simulink model "Problem8"  (R2020b)
settings: Solver=VariableStepAuto  StartTime=0.0  StopTime=inf  RelTol=1e-3
settings Model: EnablePacing=on  PacingRate=0.089000  Creator=ASUS  LastModifiedBy=ASUS

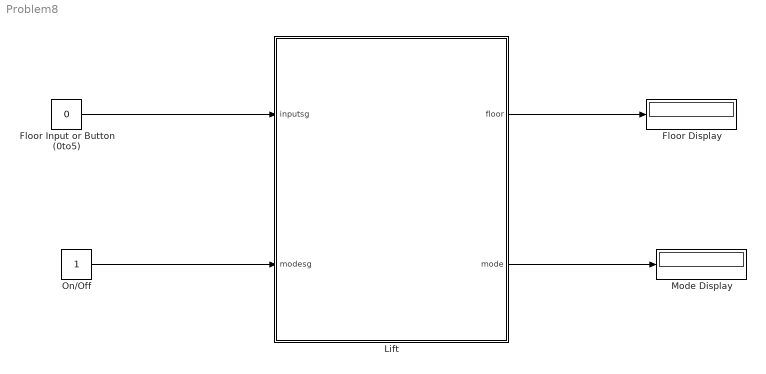
== system Problem8 ==
  Floor Display : Display
  Floor Input or Button (0to5) : Constant  Value=0
  "Lift " : Stateflow chart  TreatAsAtomicUnit=on
  Mode Display : Display
  On/Off : Constant
  wires:
  "Lift "/1(floor) -> Floor Display/1
  Floor Input or Button (0to5)/1 -> "Lift "/1(inputsg)
  "Lift "/2(mode) -> Mode Display/1
  On/Off/1 -> "Lift "/2(modesg)

== stateflow chart Problem8/Lift  ==
  state Floormovement(Floor) [function]
    (default) -> (junction 97)
    (junction 97) -> (junction 107) [order 3] : [inputsg<Floor]{send(DOWN);}
    (junction 97) -> (junction 100) [order 1] : [inputsg>Floor]{send(UP);}
    (junction 107) -> (junction 109)
    (junction 97) -> (junction 104) [order 2] : [inputsg==Floor]
    (junction 100) -> (junction 102)
    (junction 109) -> (junction 104)
    (junction 102) -> (junction 104)
    (junction 104) -> (junction 113)
  state Lift_Working_Operation [parallel]
    entry:
    mode=0;
    settings: executionOrder=1
    state LiftOn
      state Floor2
        en:
        mode=1;
        du:
        floor=2;
        Floormovement(floor);
        exit:
        mode=0
      state GroundFloor
        en:
        mode=1;
        du:
        floor=0;
        Floormovement(floor);
        exit:
        mode=0;
      state Floor1
        en:
        mode=1;
        du:
        floor=1;
        Floormovement(floor);
        exit:
        mode=0
      state Floor3
        en:
        mode=1;
        du:
        floor=3;
        Floormovement(floor);
        exit:
        mode=0
      state Floor4
        en:
        mode=1;
        du:
        floor=4;
        Floormovement(floor);
        exit:
        mode=0
      state Floor5
        en:
        mode=1;
        du:
        floor=5;
        Floormovement(floor);
        exit:
        mode=0
      (default) -> GroundFloor
      GroundFloor -> Floor1 : UP
      Floor2 -> Floor3 [order 1] : UP
      Floor1 -> Floor2 [order 1] : UP
      Floor3 -> Floor4 [order 1] : UP
      Floor4 -> Floor5 [order 1] : UP
      Floor1 -> GroundFloor [order 2] : DOWN
      Floor2 -> Floor1 [order 2] : DOWN
      Floor3 -> Floor2 [order 2] : DOWN
      Floor5 -> Floor4 : DOWN
      Floor4 -> Floor3 [order 2] : DOWN
    state LiftOff
      entry:
      mode=0;
    (default) -> LiftOn
    LiftOff -> LiftOn : [modesg==1]
    LiftOn -> LiftOff : [modesg==0]
  data: Floor function_input; inputsg input; floor output; mode output; modesg input
  events: UP local FUNCTION_CALL_EVENT; DOWN local FUNCTION_CALL_EVENT
